simulink model "SLSingleLink_End"  (R2014b)
settings: Solver=ode45  StartTime=0.0  StopTime=2*pi  MaxStep=0.05  RelTol=1e-3
PreLoadFcn:
  | g = 9.81;
  | rho = 1;
  | m = 1;
  | b = 1;
settings Model: Creator=cosorio  LastModifiedBy=cosorio
settings DataIOCC: LimitDataPoints=off  SignalLoggingSaveFormat=ModelDataLogs  SaveTime=off
settings OptimizationCC: ExpressionDepthLimit=2147483647
settings DebuggingCC: UnderspecifiedInitializationDetection=Classic  MergeDetectMultiDrivingBlocksExec=none  SolverPrmCheckMsg=none  FcnCallInpInsideContextMsg=UseLocalSettings  StateNameClashWarn=warning
settings GRTTargetCC: CombineOutputUpdateFcns=off  GRTInterface=on

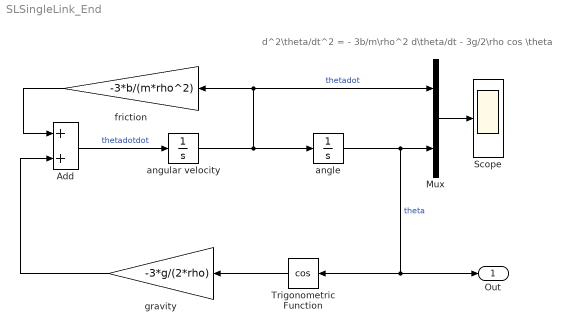
== system SLSingleLink_End ==
  note: d^2\theta/dt^2 = - 3b/m\rho^2 d\theta/dt - 3g/2\rho cos \theta
  Add : Sum
  Mux : Mux  Inputs=2
  Scope : Scope
      settings: ShowLegends=on  YMin=-8  YMax=8
  Trigonometric Function : Trigonometry  Operator=cos
  angle : Integrator  InitialCondition=45*pi/180
  angular velocity : Integrator
  friction : Gain  Gain=-3*b/(m*rho^2)
  gravity : Gain  Gain=-3*g/(2*rho)
  Out : Outport
  wires:
  angle/1 -> Trigonometric Function/1, Out/1, Mux/2  "theta"
  angular velocity/1 -> angle/1, friction/1, Mux/1  "thetadot"
  Trigonometric Function/1 -> gravity/1
  Add/1 -> angular velocity/1  "thetadotdot"
  gravity/1 -> Add/2
  friction/1 -> Add/1
  Mux/1 -> Scope/1
